simulink model "Simulink_BTL_Model_2018b"  (R2018b)
settings: Solver=ode5  StartTime=0.0  StopTime=300  FixedStep=0.001  RelTol=1e-3
settings Model: Creator=LENOVO  LastModifiedBy=LENOVO
settings DataIOCC: ReturnWorkspaceOutputs=on
settings DebuggingCC: UnconnectedInputMsg=none  UnconnectedOutputMsg=none  UnconnectedLineMsg=none
settings ModelReferenceCC: EnableRefExpFcnMdlSchedulingChecks=off
settings RTWCC: Description=Generic Real-Time Target
settings ConfigComp: CovBoundaryAbsTol=1.0e-5

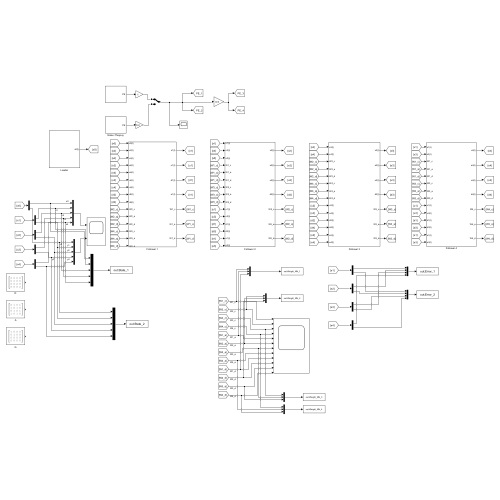
[thumbnail: Simulink's stored preview of the top-level diagram]
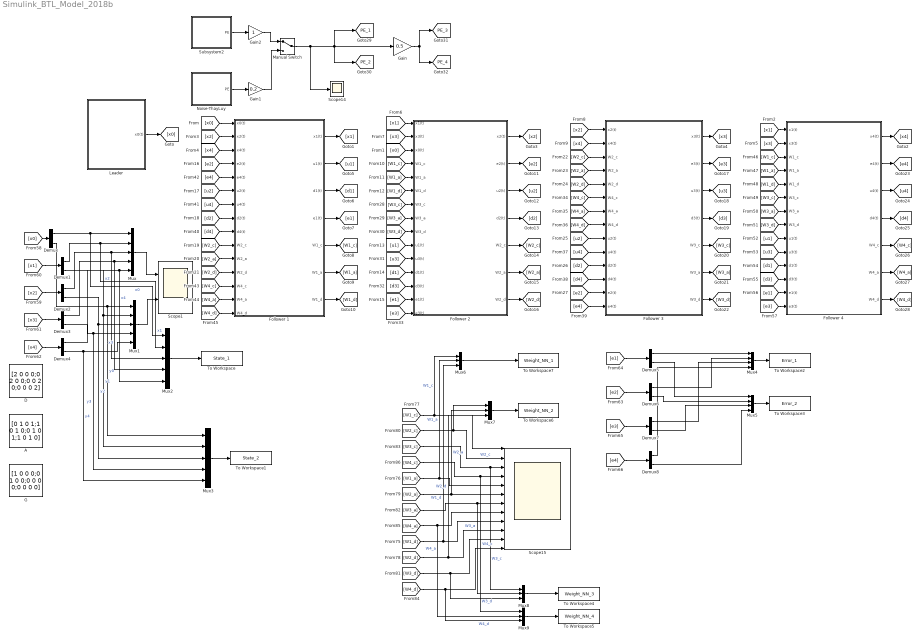
== system Simulink_BTL_Model_2018b ==
  A : Constant  Value=[0 1 0 1;1 0 1 0;0 1 0 1;1 0 1 0]
  D : Constant  Value=[2 0 0 0;0 2 0 0;0 0 2 0;0 0 0 2]
  Demux{,1..8} (9 alike) : Demux  Outputs=2
  Follower 1 : Subsystem
  Follower 2 : Subsystem
  Follower 3 : Subsystem
  Follower 4 : Subsystem
  G : Constant  Value=[1 0 0 0;0 1 0 0;0 0 0 0;0 0 0 0]
  Gain : Gain  Gain=0.5
  Gain1 : Gain  Gain=0.2
  Gain2 : Gain
  Leader : Subsystem
  Manual Switch : ManualSwitch
  Mux{,1..3} (4 alike) : Mux  Inputs=5
  Mux4 : Mux
  Mux5 : Mux
  Mux{6..9} (4 alike) : Mux  Inputs=3
  Noise-ThayLuy : Subsystem
  Scope1 : Scope  NumInputPorts=2
  Scope14 : Scope
  Scope15 : Scope  NumInputPorts=12
  Subsystem2 : Subsystem
  To Workspace : ToWorkspace  VariableName=State_1  SaveFormat=Timeseries  SampleTime=-1
  To Workspace1 : ToWorkspace  VariableName=State_2  SaveFormat=Timeseries  SampleTime=-1
  To Workspace2 : ToWorkspace  VariableName=Error_1  SaveFormat=Timeseries  SampleTime=-1
  To Workspace3 : ToWorkspace  VariableName=Error_2  SaveFormat=Timeseries  SampleTime=-1
  To Workspace4 : ToWorkspace  VariableName=Weight_NN_3  SaveFormat=Timeseries  SampleTime=-1
  To Workspace5 : ToWorkspace  VariableName=Weight_NN_4  SaveFormat=Timeseries  SampleTime=-1
  To Workspace6 : ToWorkspace  VariableName=Weight_NN_2  SaveFormat=Timeseries  SampleTime=-1
  To Workspace7 : ToWorkspace  VariableName=Weight_NN_1  SaveFormat=Timeseries  SampleTime=-1
  tag scope: PE_1=global, PE_2=global, PE_3=global, PE_4=global
  wires:
  Leader/1(x0(t)) -> [x0]
  [x0] -> Follower 1/1(x0(t))
  [x0] -> Follower 2/3(x0(t))
  Follower 1/1(x1(t)) -> [x1]
  [x1] -> Follower 4/1(x1(t))
  Follower 4/1(x4(t)) -> [x4]
  Follower 2/1(x2(t)) -> [x2]
  Follower 3/1(x3(t)) -> [x3]
  [x2] -> Follower 1/2(x2(t))
  [x4] -> Follower 1/3(x4(t))
  [x3] -> Follower 4/2(x3(t))
  [x1] -> Follower 2/1(x1(t))
  [x3] -> Follower 2/2(x3(t))
  [x2] -> Follower 3/1(x2(t))
  [x4] -> Follower 3/2(x4(t))
  Follower 1/2(u1(t)) -> [u1]
  Follower 1/3(d1(t)) -> [d1]
  Follower 1/4(e1(t)) -> [e1]
  Follower 1/5(W1_c) -> [W1_c]
  Follower 1/6(W1_a) -> [W1_a]
  Follower 1/7(W1_d) -> [W1_d]
  [W1_c] -> Follower 2/4(W1_c)
  [W1_a] -> Follower 2/5(W1_a)
  [W1_d] -> Follower 2/6(W1_d)
  [u1] -> Follower 2/10(u1(t))
  [d1] -> Follower 2/12(d1(t))
  [e1] -> Follower 2/14(e1(t))
  Follower 2/2(e2(t)) -> [e2]
  Follower 2/3(u2(t)) -> [u2]
  Follower 2/4(d2(t)) -> [d2]
  Follower 2/5(W2_c) -> [W2_c]
  Follower 2/6(W2_a) -> [W2_a]
  Follower 2/7(W2_d) -> [W2_d]
  [e2] -> Follower 1/4(e2(t))
  [u2] -> Follower 1/6(u2(t))
  [d2] -> Follower 1/8(d2(t))
  [W2_c] -> Follower 1/10(W2_c)
  [W2_a] -> Follower 1/11(W2_a)
  [W2_d] -> Follower 1/12(W2_d)
  Follower 3/2(e3(t)) -> [e3]
  Follower 3/3(u3(t)) -> [u3]
  Follower 3/4(d3(t)) -> [d3]
  Follower 3/5(W3_c) -> [W3_c]
  Follower 3/6(W3_a) -> [W3_a]
  Follower 3/7(W3_d) -> [W3_d]
  [W2_c] -> Follower 3/3(W2_c)
  [W2_a] -> Follower 3/4(W2_a)
  [W2_d] -> Follower 3/5(W2_d)
  [u2] -> Follower 3/9(u2(t))
  [d2] -> Follower 3/11(d2(t))
  [e2] -> Follower 3/13(e2(t))
  [W3_c] -> Follower 2/7(W3_c)
  [W3_a] -> Follower 2/8(W3_a)
  [W3_d] -> Follower 2/9(W3_d)
  [u3] -> Follower 2/11(u3(t))
  [d3] -> Follower 2/13(d3(t))
  [e3] -> Follower 2/15(e3(t))
  Follower 4/2(e4(t)) -> [e4]
  Follower 4/3(u4(t)) -> [u4]
  Follower 4/4(d4(t)) -> [d4]
  Follower 4/5(W4_c) -> [W4_c]
  Follower 4/6(W4_a) -> [W4_a]
  Follower 4/7(W4_d) -> [W4_d]
  [W4_c] -> Follower 3/6(W4_c)
  [W4_a] -> Follower 3/7(W4_a)
  [W4_d] -> Follower 3/8(W4_d)
  [u4] -> Follower 3/10(u4(t))
  [d4] -> Follower 3/12(d4(t))
  [e4] -> Follower 3/14(e4(t))
  [d4] -> Follower 1/9(d4(t))
  [u4] -> Follower 1/7(u4(t))
  [e4] -> Follower 1/5(e4(t))
  [W4_c] -> Follower 1/13(W4_c)
  [W4_a] -> Follower 1/14(W4_a)
  [W4_d] -> Follower 1/15(W4_d)
  [W1_c] -> Follower 4/3(W1_c)
  [W1_a] -> Follower 4/4(W1_a)
  [W1_d] -> Follower 4/5(W1_d)
  [W3_c] -> Follower 4/6(W3_c)
  [W3_a] -> Follower 4/7(W3_a)
  [W3_d] -> Follower 4/8(W3_d)
  [u1] -> Follower 4/9(u1(t))
  [u3] -> Follower 4/10(u3(t))
  [d1] -> Follower 4/11(d1(t))
  [d3] -> Follower 4/12(d3(t))
  [e1] -> Follower 4/13(e1(t))
  [e3] -> Follower 4/14(e3(t))
  [x0] -> Demux/1
  [x1] -> Demux1/1
  [x2] -> Demux2/1
  [x3] -> Demux3/1
  [x4] -> Demux4/1
  Demux/1 -> Mux2/1, Mux/1  "x0"
  Demux1/1 -> Mux2/2, Mux/2  "x1"
  Demux2/1 -> Mux2/3, Mux/3  "x2"
  Demux3/1 -> Mux2/4, Mux/4  "x3"
  Demux4/1 -> Mux2/5, Mux/5  "x4"
  Demux/2 -> Mux3/1, Mux1/1  "y0"
  Demux1/2 -> Mux3/2, Mux1/2  "y1"
  Demux2/2 -> Mux3/3, Mux1/3  "y2"
  Demux3/2 -> Mux3/4, Mux1/4  "y3"
  Demux4/2 -> Mux3/5, Mux1/5  "y4"
  Subsystem2/1(PE) -> Gain2/1
  Gain/1 -> [PE_3], [PE_4]
  Noise-ThayLuy/1(PE) -> Gain1/1
  Manual Switch/1 -> Scope14/1, [PE_1], Gain/1, [PE_2]
  Gain1/1 -> Manual Switch/2
  Gain2/1 -> Manual Switch/1
  [W1_c] -> Mux6/1, Scope15/1  "W1_c"
  [W2_c] -> Mux7/1, Scope15/2  "W2_c"
  [W3_c] -> Mux8/1, Scope15/3  "W3_c"
  [W4_c] -> Mux9/1, Scope15/4  "W4_c"
  [W1_a] -> Mux6/2, Scope15/5  "W1_a"
  [W2_a] -> Mux7/2, Scope15/6  "W2_a"
  [W3_a] -> Mux8/2, Scope15/7  "W3_a"
  [W4_a] -> Mux9/2, Scope15/8  "W4_a"
  [W1_d] -> Mux6/3, Scope15/9  "W1_d"
  [W2_d] -> Scope15/10, Mux7/3  "W2_d"
  [W3_d] -> Mux8/3, Scope15/11  "W3_d"
  [W4_d] -> Mux9/3, Scope15/12  "W4_d"
  Mux/1 -> Scope1/1
  Mux1/1 -> Scope1/2
  Mux2/1 -> To Workspace/1
  Mux3/1 -> To Workspace1/1
  [e1] -> Demux5/1
  [e2] -> Demux6/1
  [e3] -> Demux7/1
  [e4] -> Demux8/1
  Demux5/1 -> Mux4/1
  Demux6/1 -> Mux4/2
  Demux7/1 -> Mux4/3
  Demux8/1 -> Mux4/4
  Demux5/2 -> Mux5/1
  Demux6/2 -> Mux5/2
  Demux7/2 -> Mux5/3
  Demux8/2 -> Mux5/4
  Mux4/1 -> To Workspace2/1
  Mux5/1 -> To Workspace3/1
  Mux8/1 -> To Workspace4/1
  Mux9/1 -> To Workspace5/1
  Mux7/1 -> To Workspace6/1
  Mux6/1 -> To Workspace7/1

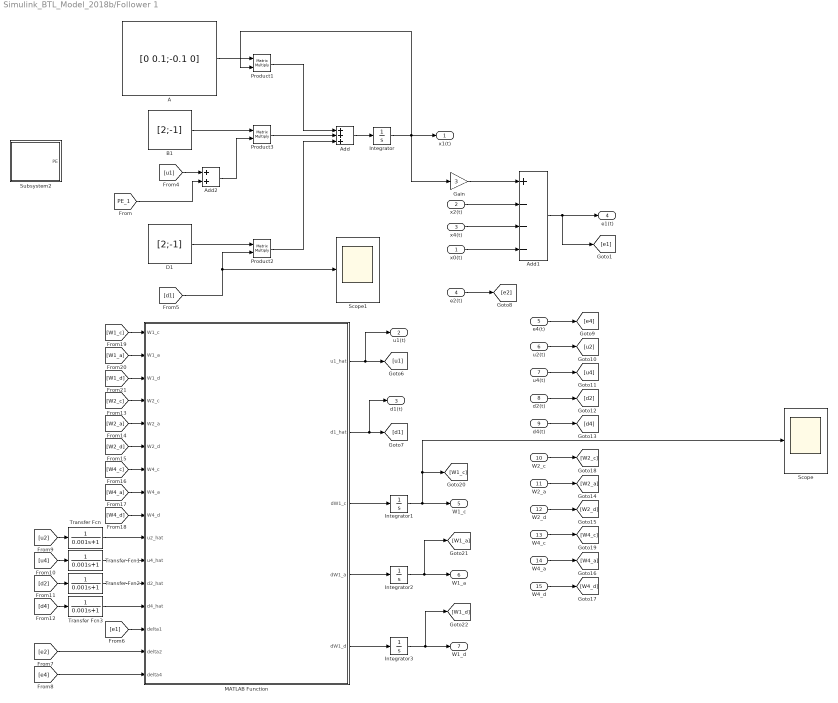
== system Simulink_BTL_Model_2018b/Follower 1 ==
  x0(t) : Inport
  x2(t) : Inport  Port=2
  x4(t) : Inport  Port=3
  e2(t) : Inport  Port=4
  e4(t) : Inport  Port=5
  u2(t) : Inport  Port=6
  u4(t) : Inport  Port=7
  d2(t) : Inport  Port=8
  d4(t) : Inport  Port=9
  W2_c : Inport  Port=10
  W2_a : Inport  Port=11
  W2_d : Inport  Port=12
  W4_c : Inport  Port=13
  W4_a : Inport  Port=14
  W4_d : Inport  Port=15
  A : Constant  Value=[0 0.1;-0.1 0]
  Add : Sum  Inputs=+++
  Add1 : Sum  Inputs=+---
  Add2 : Sum
  B1 : Constant  Value=[2;-1]  VectorParams1D=off
  D1 : Constant  Value=[2;-1]  VectorParams1D=off
  Gain : Gain  Gain=3
  Integrator : Integrator  InitialCondition=[1;0]
  Integrator1 : Integrator
  Integrator2 : Integrator
  Integrator3 : Integrator
  MATLAB Function : MATLAB Function  TreatAsAtomicUnit=on
  Product1 : Product  Multiplication=Matrix(*)
  Product2 : Product  Multiplication=Matrix(*)
  Product3 : Product  Multiplication=Matrix(*)
  Scope : Scope
  Scope1 : Scope
  Subsystem2 : Subsystem
  Transfer Fcn{,1..3} (4 alike) : TransferFcn  Denominator=[0.001 1]
  x1(t) : Outport
  u1(t) : Outport  Port=2
  d1(t) : Outport  Port=3
  e1(t) : Outport  Port=4
  W1_c : Outport  Port=5
  W1_a : Outport  Port=6
  W1_d : Outport  Port=7
  wires:
  A/1 -> Product1/1
  Product1/1 -> Add/1
  D1/1 -> Product2/1
  Add/1 -> Integrator/1
  Integrator/1 -> Gain/1, Product1/2, x1(t)/1
  B1/1 -> Product3/1
  Product3/1 -> Add/2
  Product2/1 -> Add/3
  x2(t)/1 -> Add1/2
  x4(t)/1 -> Add1/3
  x0(t)/1 -> Add1/4
  Gain/1 -> Add1/1
  Add1/1 -> [e1], e1(t)/1
  MATLAB Function/3(dW1_c) -> Integrator1/1
  MATLAB Function/4(dW1_a) -> Integrator2/1
  MATLAB Function/5(dW1_d) -> Integrator3/1
  MATLAB Function/1(u1_hat) -> u1(t)/1, [u1]
  MATLAB Function/2(d1_hat) -> d1(t)/1, [d1]
  [d1] -> Scope1/1, Product2/2
  [u1] -> Add2/1
  Add2/1 -> Product3/2
  [e1] -> MATLAB Function/14(delta1)
  e2(t)/1 -> [e2]
  e4(t)/1 -> [e4]
  u2(t)/1 -> [u2]
  u4(t)/1 -> [u4]
  d2(t)/1 -> [d2]
  d4(t)/1 -> [d4]
  [u2] -> Transfer Fcn/1
  [u4] -> Transfer Fcn1/1
  [d2] -> Transfer Fcn2/1
  [d4] -> Transfer Fcn3/1
  W2_d/1 -> [W2_d]
  W2_a/1 -> [W2_a]
  W2_c/1 -> [W2_c]
  W4_a/1 -> [W4_a]
  W4_c/1 -> [W4_c]
  W4_d/1 -> [W4_d]
  [W2_c] -> MATLAB Function/4(W2_c)
  [W2_a] -> MATLAB Function/5(W2_a)
  [W2_d] -> MATLAB Function/6(W2_d)
  [W4_c] -> MATLAB Function/7(W4_c)
  [W4_a] -> MATLAB Function/8(W4_a)
  [W4_d] -> MATLAB Function/9(W4_d)
  Integrator1/1 -> Scope/1, [W1_c], W1_c/1
  Integrator2/1 -> [W1_a], W1_a/1
  Integrator3/1 -> [W1_d], W1_d/1
  [W1_c] -> MATLAB Function/1(W1_c)
  [W1_a] -> MATLAB Function/2(W1_a)
  [W1_d] -> MATLAB Function/3(W1_d)
  Transfer Fcn/1 -> MATLAB Function/10(u2_hat)
  Transfer Fcn1/1 -> MATLAB Function/11(u4_hat)
  Transfer Fcn2/1 -> MATLAB Function/12(d2_hat)
  Transfer Fcn3/1 -> MATLAB Function/13(d4_hat)
  [e2] -> MATLAB Function/15(delta2)
  [e4] -> MATLAB Function/16(delta4)
  [PE_1] -> Add2/2

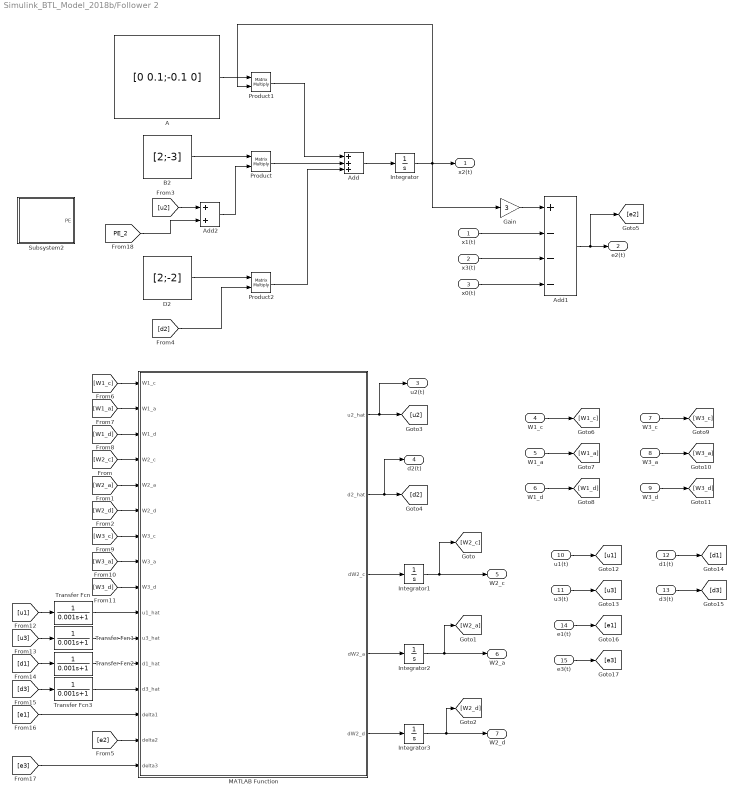
== system Simulink_BTL_Model_2018b/Follower 2 ==
  x1(t) : Inport
  x3(t) : Inport  Port=2
  x0(t) : Inport  Port=3
  W1_c : Inport  Port=4
  W1_a : Inport  Port=5
  W1_d : Inport  Port=6
  W3_c : Inport  Port=7
  W3_a : Inport  Port=8
  W3_d : Inport  Port=9
  u1(t) : Inport  Port=10
  u3(t) : Inport  Port=11
  d1(t) : Inport  Port=12
  d3(t) : Inport  Port=13
  e1(t) : Inport  Port=14
  e3(t) : Inport  Port=15
  A : Constant  Value=[0 0.1;-0.1 0]
  Add : Sum  Inputs=+++
  Add1 : Sum  Inputs=+---
  Add2 : Sum
  B2 : Constant  Value=[2;-3]  VectorParams1D=off
  D2 : Constant  Value=[2;-2]  VectorParams1D=off
  Gain : Gain  Gain=3
  Integrator : Integrator  InitialCondition=[1;0]
  Integrator1 : Integrator
  Integrator2 : Integrator
  Integrator3 : Integrator
  MATLAB Function : MATLAB Function  TreatAsAtomicUnit=on
  Product : Product  Multiplication=Matrix(*)
  Product1 : Product  Multiplication=Matrix(*)
  Product2 : Product  Multiplication=Matrix(*)
  Subsystem2 : Subsystem
  Transfer Fcn{,1..3} (4 alike) : TransferFcn  Denominator=[0.001 1]
  x2(t) : Outport
  e2(t) : Outport  Port=2
  u2(t) : Outport  Port=3
  d2(t) : Outport  Port=4
  W2_c : Outport  Port=5
  W2_a : Outport  Port=6
  W2_d : Outport  Port=7
  wires:
  Integrator/1 -> Gain/1, x2(t)/1, Product1/2
  Product1/1 -> Add/1
  Add/1 -> Integrator/1
  B2/1 -> Product/1
  A/1 -> Product1/1
  Product/1 -> Add/2
  D2/1 -> Product2/1
  Product2/1 -> Add/3
  Add1/1 -> [e2], e2(t)/1
  x1(t)/1 -> Add1/2
  x3(t)/1 -> Add1/3
  x0(t)/1 -> Add1/4
  Gain/1 -> Add1/1
  MATLAB Function/3(dW2_c) -> Integrator1/1
  MATLAB Function/4(dW2_a) -> Integrator2/1
  MATLAB Function/5(dW2_d) -> Integrator3/1
  Integrator1/1 -> W2_c/1, [W2_c]
  [W2_c] -> MATLAB Function/4(W2_c)
  Integrator2/1 -> W2_a/1, [W2_a]
  [W2_a] -> MATLAB Function/5(W2_a)
  [W2_d] -> MATLAB Function/6(W2_d)
  Integrator3/1 -> [W2_d], W2_d/1
  MATLAB Function/1(u2_hat) -> u2(t)/1, [u2]
  MATLAB Function/2(d2_hat) -> d2(t)/1, [d2]
  [u2] -> Add2/1
  Add2/1 -> Product/2
  [d2] -> Product2/2
  [e2] -> MATLAB Function/15(delta2)
  W1_c/1 -> [W1_c]
  W1_a/1 -> [W1_a]
  W1_d/1 -> [W1_d]
  W3_d/1 -> [W3_d]
  W3_c/1 -> [W3_c]
  W3_a/1 -> [W3_a]
  u1(t)/1 -> [u1]
  u3(t)/1 -> [u3]
  d3(t)/1 -> [d3]
  d1(t)/1 -> [d1]
  e1(t)/1 -> [e1]
  e3(t)/1 -> [e3]
  [W1_c] -> MATLAB Function/1(W1_c)
  [W1_d] -> MATLAB Function/3(W1_d)
  [W3_c] -> MATLAB Function/7(W3_c)
  [W3_a] -> MATLAB Function/8(W3_a)
  [W3_d] -> MATLAB Function/9(W3_d)
  [u1] -> Transfer Fcn/1
  [u3] -> Transfer Fcn1/1
  [d1] -> Transfer Fcn2/1
  [W1_a] -> MATLAB Function/2(W1_a)
  [d3] -> Transfer Fcn3/1
  Transfer Fcn/1 -> MATLAB Function/10(u1_hat)
  Transfer Fcn1/1 -> MATLAB Function/11(u3_hat)
  Transfer Fcn2/1 -> MATLAB Function/12(d1_hat)
  Transfer Fcn3/1 -> MATLAB Function/13(d3_hat)
  [e1] -> MATLAB Function/14(delta1)
  [e3] -> MATLAB Function/16(delta3)
  [PE_2] -> Add2/2

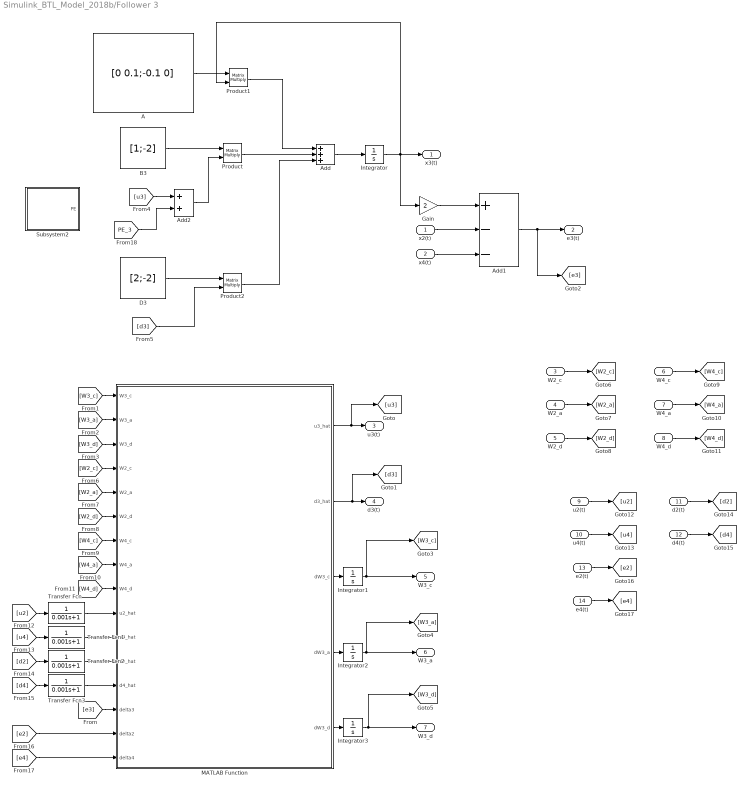
== system Simulink_BTL_Model_2018b/Follower 3 ==
  x2(t) : Inport
  x4(t) : Inport  Port=2
  W2_c : Inport  Port=3
  W2_a : Inport  Port=4
  W2_d : Inport  Port=5
  W4_c : Inport  Port=6
  W4_a : Inport  Port=7
  W4_d : Inport  Port=8
  u2(t) : Inport  Port=9
  u4(t) : Inport  Port=10
  d2(t) : Inport  Port=11
  d4(t) : Inport  Port=12
  e2(t) : Inport  Port=13
  e4(t) : Inport  Port=14
  A : Constant  Value=[0 0.1;-0.1 0]
  Add : Sum  Inputs=+++
  Add1 : Sum  Inputs=+--
  Add2 : Sum
  B3 : Constant  Value=[1;-2]  VectorParams1D=off
  D3 : Constant  Value=[2;-2]  VectorParams1D=off
  Gain : Gain  Gain=2
  Integrator : Integrator  InitialCondition=[1;0]
  Integrator1 : Integrator
  Integrator2 : Integrator
  Integrator3 : Integrator
  MATLAB Function : MATLAB Function  TreatAsAtomicUnit=on
  Product : Product  Multiplication=Matrix(*)
  Product1 : Product  Multiplication=Matrix(*)
  Product2 : Product  Multiplication=Matrix(*)
  Subsystem2 : Subsystem
  Transfer Fcn{,1..3} (4 alike) : TransferFcn  Denominator=[0.001 1]
  x3(t) : Outport
  e3(t) : Outport  Port=2
  u3(t) : Outport  Port=3
  d3(t) : Outport  Port=4
  W3_c : Outport  Port=5
  W3_a : Outport  Port=6
  W3_d : Outport  Port=7
  wires:
  Integrator/1 -> Gain/1, x3(t)/1, Product1/2
  Product1/1 -> Add/1
  Add/1 -> Integrator/1
  B3/1 -> Product/1
  A/1 -> Product1/1
  Product/1 -> Add/2
  D3/1 -> Product2/1
  Product2/1 -> Add/3
  x2(t)/1 -> Add1/2
  Gain/1 -> Add1/1
  x4(t)/1 -> Add1/3
  Add1/1 -> [e3], e3(t)/1
  MATLAB Function/1(u3_hat) -> [u3], u3(t)/1
  MATLAB Function/2(d3_hat) -> d3(t)/1, [d3]
  MATLAB Function/3(dW3_c) -> Integrator1/1
  MATLAB Function/4(dW3_a) -> Integrator2/1
  MATLAB Function/5(dW3_d) -> Integrator3/1
  [e3] -> MATLAB Function/14(delta3)
  [W3_c] -> MATLAB Function/1(W3_c)
  [W3_a] -> MATLAB Function/2(W3_a)
  [W3_d] -> MATLAB Function/3(W3_d)
  [u3] -> Add2/1
  Add2/1 -> Product/2
  [d3] -> Product2/2
  e2(t)/1 -> [e2]
  W4_c/1 -> [W4_c]
  W4_d/1 -> [W4_d]
  W4_a/1 -> [W4_a]
  W2_d/1 -> [W2_d]
  u2(t)/1 -> [u2]
  W2_c/1 -> [W2_c]
  W2_a/1 -> [W2_a]
  d4(t)/1 -> [d4]
  d2(t)/1 -> [d2]
  e4(t)/1 -> [e4]
  u4(t)/1 -> [u4]
  [W2_c] -> MATLAB Function/4(W2_c)
  [W2_a] -> MATLAB Function/5(W2_a)
  [W2_d] -> MATLAB Function/6(W2_d)
  [W4_c] -> MATLAB Function/7(W4_c)
  [W4_a] -> MATLAB Function/8(W4_a)
  [W4_d] -> MATLAB Function/9(W4_d)
  [u2] -> Transfer Fcn/1
  [u4] -> Transfer Fcn1/1
  [d2] -> Transfer Fcn2/1
  [d4] -> Transfer Fcn3/1
  Transfer Fcn/1 -> MATLAB Function/10(u2_hat)
  Transfer Fcn1/1 -> MATLAB Function/11(u4_hat)
  Transfer Fcn2/1 -> MATLAB Function/12(d2_hat)
  Transfer Fcn3/1 -> MATLAB Function/13(d4_hat)
  [e2] -> MATLAB Function/15(delta2)
  [e4] -> MATLAB Function/16(delta4)
  Integrator1/1 -> [W3_c], W3_c/1
  Integrator2/1 -> [W3_a], W3_a/1
  Integrator3/1 -> [W3_d], W3_d/1
  [PE_3] -> Add2/2

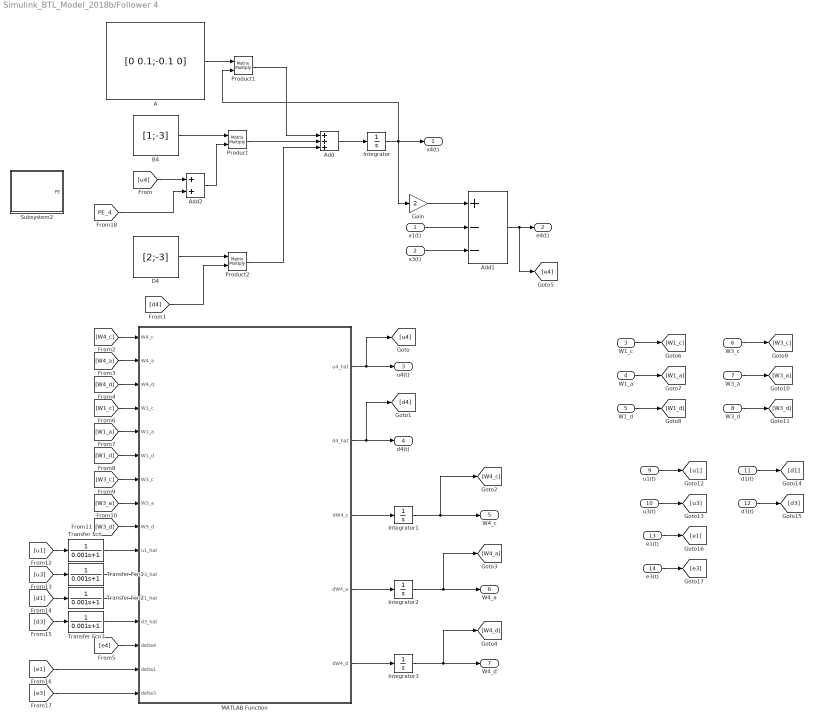
== system Simulink_BTL_Model_2018b/Follower 4 ==
  x1(t) : Inport
  x3(t) : Inport  Port=2
  W1_c : Inport  Port=3
  W1_a : Inport  Port=4
  W1_d : Inport  Port=5
  W3_c : Inport  Port=6
  W3_a : Inport  Port=7
  W3_d : Inport  Port=8
  u1(t) : Inport  Port=9
  u3(t) : Inport  Port=10
  d1(t) : Inport  Port=11
  d3(t) : Inport  Port=12
  e1(t) : Inport  Port=13
  e3(t) : Inport  Port=14
  A : Constant  Value=[0 0.1;-0.1 0]
  Add : Sum  Inputs=+++
  Add1 : Sum  Inputs=+--
  Add2 : Sum
  B4 : Constant  Value=[1;-3]  VectorParams1D=off
  D4 : Constant  Value=[2;-3]  VectorParams1D=off
  Gain : Gain  Gain=2
  Integrator : Integrator  InitialCondition=[1;0]
  Integrator1 : Integrator
  Integrator2 : Integrator
  Integrator3 : Integrator
  MATLAB Function : MATLAB Function  TreatAsAtomicUnit=on
  Product : Product  Multiplication=Matrix(*)
  Product1 : Product  Multiplication=Matrix(*)
  Product2 : Product  Multiplication=Matrix(*)
  Subsystem2 : Subsystem
  Transfer Fcn{,1..3} (4 alike) : TransferFcn  Denominator=[0.001 1]
  x4(t) : Outport
  e4(t) : Outport  Port=2
  u4(t) : Outport  Port=3
  d4(t) : Outport  Port=4
  W4_c : Outport  Port=5
  W4_a : Outport  Port=6
  W4_d : Outport  Port=7
  wires:
  Product1/1 -> Add/1
  B4/1 -> Product/1
  A/1 -> Product1/1
  Product/1 -> Add/2
  D4/1 -> Product2/1
  Product2/1 -> Add/3
  Add/1 -> Integrator/1
  Integrator/1 -> Product1/2, Gain/1, x4(t)/1
  Add1/1 -> [e4], e4(t)/1
  x1(t)/1 -> Add1/2
  x3(t)/1 -> Add1/3
  Gain/1 -> Add1/1
  MATLAB Function/1(u4_hat) -> [u4], u4(t)/1
  MATLAB Function/2(d4_hat) -> [d4], d4(t)/1
  [u4] -> Add2/1
  [d4] -> Product2/2
  MATLAB Function/3(dW4_c) -> Integrator1/1
  MATLAB Function/4(dW4_a) -> Integrator2/1
  MATLAB Function/5(dW4_d) -> Integrator3/1
  Integrator1/1 -> [W4_c], W4_c/1
  Integrator2/1 -> [W4_a], W4_a/1
  Integrator3/1 -> [W4_d], W4_d/1
  [W4_c] -> MATLAB Function/1(W4_c)
  [W4_a] -> MATLAB Function/2(W4_a)
  [W4_d] -> MATLAB Function/3(W4_d)
  [e4] -> MATLAB Function/14(delta4)
  u3(t)/1 -> [u3]
  e3(t)/1 -> [e3]
  d1(t)/1 -> [d1]
  W1_c/1 -> [W1_c]
  u1(t)/1 -> [u1]
  d3(t)/1 -> [d3]
  W1_a/1 -> [W1_a]
  W3_a/1 -> [W3_a]
  W3_c/1 -> [W3_c]
  e1(t)/1 -> [e1]
  W3_d/1 -> [W3_d]
  W1_d/1 -> [W1_d]
  [W1_c] -> MATLAB Function/4(W1_c)
  [W1_a] -> MATLAB Function/5(W1_a)
  [W1_d] -> MATLAB Function/6(W1_d)
  [W3_c] -> MATLAB Function/7(W3_c)
  [W3_a] -> MATLAB Function/8(W3_a)
  [W3_d] -> MATLAB Function/9(W3_d)
  [u1] -> Transfer Fcn/1
  [u3] -> Transfer Fcn1/1
  [d1] -> Transfer Fcn2/1
  [d3] -> Transfer Fcn3/1
  Add2/1 -> Product/2
  Transfer Fcn/1 -> MATLAB Function/10(u1_hat)
  Transfer Fcn1/1 -> MATLAB Function/11(u3_hat)
  Transfer Fcn2/1 -> MATLAB Function/12(d1_hat)
  Transfer Fcn3/1 -> MATLAB Function/13(d3_hat)
  [e1] -> MATLAB Function/15(delta1)
  [e3] -> MATLAB Function/16(delta3)
  [PE_4] -> Add2/2

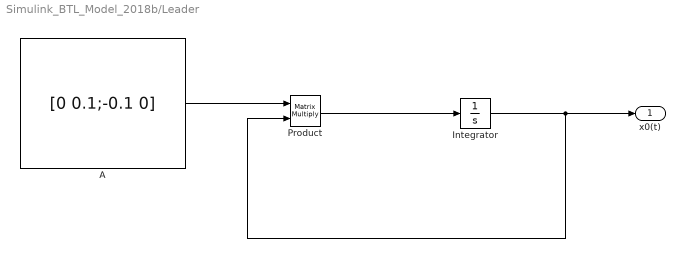
== system Simulink_BTL_Model_2018b/Leader ==
  A : Constant  Value=[0 0.1;-0.1 0]
  Integrator : Integrator  InitialCondition=[1;0]
  Product : Product  Multiplication=Matrix(*)
  x0(t) : Outport
  wires:
  Product/1 -> Integrator/1
  A/1 -> Product/1
  Integrator/1 -> x0(t)/1, Product/2

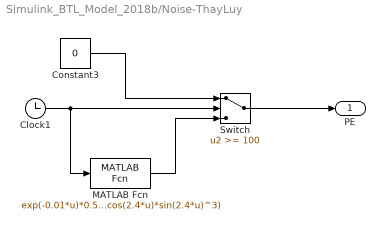
== system Simulink_BTL_Model_2018b/Noise-ThayLuy ==
  Clock1 : Clock
  Constant3 : Constant  Value=0
  MATLAB Fcn : MATLABFcn  MATLABFcn=exp(-0.01*u)*0.5*(sin(u)^2*cos(u)+sin(2*u)^2*cos(0.1*u)+sin(-1.2*u)^2*cos(0.5*u)+sin(u)^5+sin(1.12*u)^2+cos(2.4*u)*sin(2.4*u)^3)
  Switch : Switch  Threshold=100
  PE : Outport
  wires:
  Constant3/1 -> Switch/1
  Clock1/1 -> Switch/2, MATLAB Fcn/1
  MATLAB Fcn/1 -> Switch/3
  Switch/1 -> PE/1

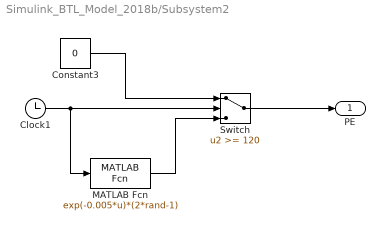
== system Simulink_BTL_Model_2018b/Subsystem2 ==
  Clock1 : Clock
  Constant3 : Constant  Value=0
  MATLAB Fcn : MATLABFcn  MATLABFcn=exp(-0.005*u)*(2*rand-1)
  Switch : Switch  Threshold=120
  PE : Outport
  wires:
  Constant3/1 -> Switch/1
  Clock1/1 -> Switch/2, MATLAB Fcn/1
  MATLAB Fcn/1 -> Switch/3
  Switch/1 -> PE/1

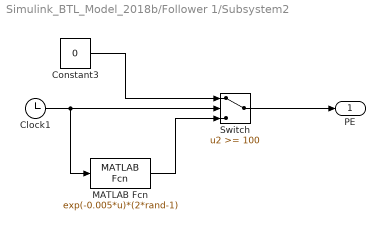
== system Simulink_BTL_Model_2018b/Follower 1/Subsystem2 ==
  Clock1 : Clock
  Constant3 : Constant  Value=0
  MATLAB Fcn : MATLABFcn  MATLABFcn=exp(-0.005*u)*(2*rand-1)
  Switch : Switch  Threshold=100
  PE : Outport
  wires:
  Constant3/1 -> Switch/1
  Clock1/1 -> Switch/2, MATLAB Fcn/1
  MATLAB Fcn/1 -> Switch/3
  Switch/1 -> PE/1

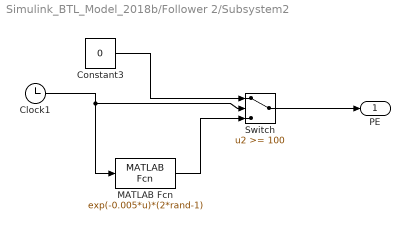
== system Simulink_BTL_Model_2018b/Follower 2/Subsystem2 ==
  Clock1 : Clock
  Constant3 : Constant  Value=0
  MATLAB Fcn : MATLABFcn  MATLABFcn=exp(-0.005*u)*(2*rand-1)
  Switch : Switch  Threshold=100
  PE : Outport
  wires:
  Constant3/1 -> Switch/1
  Clock1/1 -> Switch/2, MATLAB Fcn/1
  MATLAB Fcn/1 -> Switch/3
  Switch/1 -> PE/1

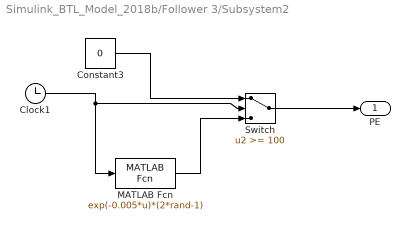
== system Simulink_BTL_Model_2018b/Follower 3/Subsystem2 ==
  Clock1 : Clock
  Constant3 : Constant  Value=0
  MATLAB Fcn : MATLABFcn  MATLABFcn=exp(-0.005*u)*(2*rand-1)
  Switch : Switch  Threshold=100
  PE : Outport
  wires:
  Constant3/1 -> Switch/1
  Clock1/1 -> Switch/2, MATLAB Fcn/1
  MATLAB Fcn/1 -> Switch/3
  Switch/1 -> PE/1

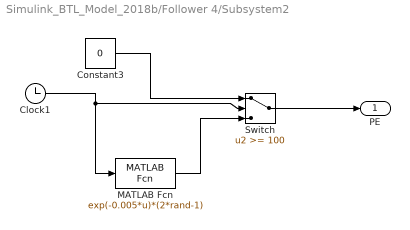
== system Simulink_BTL_Model_2018b/Follower 4/Subsystem2 ==
  Clock1 : Clock
  Constant3 : Constant  Value=0
  MATLAB Fcn : MATLABFcn  MATLABFcn=exp(-0.005*u)*(2*rand-1)
  Switch : Switch  Threshold=100
  PE : Outport
  wires:
  Constant3/1 -> Switch/1
  Clock1/1 -> Switch/2, MATLAB Fcn/1
  MATLAB Fcn/1 -> Switch/3
  Switch/1 -> PE/1

== matlab function Simulink_BTL_Model_2018b/Follower 2/MATLAB Function ==
  data: u2_hat output; W1_c input; W1_a input; W1_d input; W2_c input; W2_a input; W2_d input; W3_c input; W3_a input; W3_d input; u1_hat input; u3_hat input; d1_hat input; d3_hat input; delta1 input; delta2 input; delta3 input; d2_hat output; dW2_c output; dW2_a output; dW2_d output
function [u2_hat, d2_hat, dW2_c, dW2_a, dW2_d] = Follower2_Controller( W1_c, W1_a, W1_d, W2_c, W2_a, W2_d, W3_c, W3_a, W3_d, u1_hat, u3_hat, d1_hat, d3_hat,delta1, delta2, delta3)
    % CÁC BIẾN ĐẦU VÀO TỪ SIMULINK:
    % x1, x0, x2, x4: Trạng thái của bản thân, leader và hàng xóm (2x1)
    % W1_*, W2_*, W4_*: Trọng số của 3 mạng NNs của bản thân và hàng xóm (3x1)
    % u1_hat, u3_hat, d1_hat, d3_hat: Tín hiệu điều khiển/nhiễu của hàng xóm (1x1)
    % delta1, delta3: Sai số bám sát của hàng xóm (2x1)
    u2_hat = zeros(1,1);
    d2_hat = zeros(1,1);
    dW2_c = zeros(3,1);
    dW2_a = zeros(3,1);
    dW2_d = zeros(3,1);
    %% 1. KHỞI TẠO THÔNG SỐ HỆ THỐNG VÀ ĐỒ THỊ (Hardcode cho Node 1)
    % Đồ thị: N1 = {1, 3}
    d1 = 2; g1 = 1;
    d2 = 2; g2 = 1;
    d3 = 2; g3 = 0;
    
    gamma = 1; % Hệ số L2-gain (thay đổi theo thiết kế của bạn)
    
    % Ma trận động học (Ví dụ theo bài báo, hãy thay số thực tế của bạn)
    A  = [0 0.1; -0.1 0]; 
    B1 = [2; -1]; D1 = [2; -1];
    B2 = [2; -3]; D2 = [2; -2];
    B3 = [1; -2]; D3 = [2; -2];
    
    % Ma trận trọng số chi phí (Q, R, T)
    Q22 = eye(2);
    R22 = 1; T22 = 1;
    R21 = 1; T21 = 1; % Trọng số cho u1, d1 trong hàm mục tiêu của 1
    R23 = 1; T23 = 1; % Trọng số cho u3, d3 trong hàm mục tiêu của 1
    
    R11 = 1; T11 = 1; % Của node 1
    R33 = 1; T33 = 1; % Của node 3
    
    % Tốc độ học (Learning rates) và tham số mạng NNs
    a2 = 0.005; a2_a = 0.007; a2_d = 0.005;
    S2 = 10; F2 = 10; S_bar2 = 10; F_bar2 = 10;

    % Hàm tính ma trận đạo hàm 3x2
    dphi_1 = [2*delta1(1), 0; 
              delta1(2), delta1(1); 
              0, 2*delta1(2)];
          
    dphi_2 = [2*delta2(1), 0; 
              delta2(2), delta2(1); 
              0, 2*delta2(2)];
          
    dphi_3 = [2*delta3(1), 0; 
              delta3(2), delta3(1); 
              0, 2*delta3(2)];

    %% 3. TÍNH TÍN HIỆU ĐẦU RA ACTOR & DISTURBANCE (Eq 55, 56)
    % Tính tín hiệu u1, v1 dự kiến dựa trên trọng số hiện tại
    u2_hat = -(d2 + g2) * (1/R22) * B2' * dphi_2' * W2_a;
    d2_hat = (1/gamma^2) * (d2 + g2) * (1/T22) * D2' * dphi_2' * W2_d;

    %% 4. TÍNH TOÁN CÁC BIẾN TRUNG GIAN
    % D_bar và E_bar (3x3)
    D_bar2 = dphi_2 * B2 * (1/R22) * B2' * dphi_2';
    E_bar2 = dphi_2 * D2 * (1/T22) * D2' * dphi_2';
    
    % Tính sigma_{i+N} (Lưu ý: dùng u_hat, v_hat theo đúng lý thuyết)
    % sigma_2_N = dphi_2 * (A * delta2 + (d2 + g2)*B2*u3_hat - (B3*u3_hat + B1*u1_hat) ...
    %                       + (d2 + g2)*D2*d3_hat - (D3*d3_hat + D1*d1_hat));

    sigma_2_N = dphi_2 * (A * delta2 + (d2 + g2)*B2*u2_hat - (B3*u3_hat + B1*u1_hat) ...
                          + (d2 + g2)*D2*d2_hat - (D3*d3_hat + D1*d1_hat));
                      
    m_s2 = (sigma_2_N' * sigma_2_N) + 1;
    sigma_bar_2_N = sigma_2_N / m_s2; % Vector 3x1

    %% 5. TÍNH TỔNG TỪ CÁC HÀNG XÓM (Node 2 và Node 4)
    % -- Của Node 1 --
    term_B1 = dphi_1 * B1 * (1/R11) * R21 * (1/R11) * B1' * dphi_1';
    term_D1 = dphi_1 * D1 * (1/T11) * T21 * (1/T11) * D1' * dphi_1';
    
    sum57_a_1 = (d1 + g1)^2 * W1_a' * term_B1 * W1_a;
    sum57_d_1 = (d1 + g1)^2 * W1_d' * term_D1 * W1_d;
    sum58_a_1 = (d1 + g1)^2 * term_B1 * W1_a .* (sigma_bar_2_N' * W1_c / m_s2);
    sum59_d_1 = (d1 + g1)^2 * term_D1 * W1_d .* (sigma_bar_2_N' * W1_c / m_s2);
    
    % -- Của Node 3 --
    term_B3 = dphi_3 * B3 * (1/R33) * R23 * (1/R33) * B3' * dphi_3';
    term_D3 = dphi_3 * D3 * (1/T33) * T23 * (1/T33) * D3' * dphi_3';
    
    sum57_a_3 = (d3 + g3)^2 * W3_a' * term_B3 * W3_a;
    sum57_d_3 = (d3 + g3)^2 * W3_d' * term_D3 * W3_d;
    sum58_a_3 = (d3 + g3)^2 * term_B3 * W3_a .* (sigma_bar_2_N' * W3_c / m_s2);
    sum59_d_3 = (d3 + g3)^2 * term_D3 * W3_d .* (sigma_bar_2_N' * W3_c / m_s2);
    
    % Gộp tổng
    sum57_actor = sum57_a_1 + sum57_a_3; % Vô hướng
    sum57_dist  = sum57_d_1 + sum57_d_3; % Vô hướng
    sum58_actor = sum58_a_1 + sum58_a_3; % Vector 3x1
    sum59_dist  = sum59_d_1 + sum59_d_3; % Vector 3x1

    %% 6. LUẬT CẬP NHẬT TRỌNG SỐ (Equations 57, 58, 59)
    % 6.1 Critic
    term1_57 = sigma_2_N' * W2_c + 0.5 * delta2' * Q22 * delta2;
    term2_57 = 0.5 * (d2 + g2)^2 * W2_a' * D_bar2 * W2_a;
    term3_57 = - (1 / (2 * gamma^2)) * (d2 + g2)^2 * W2_d' * E_bar2 * W2_d;
    term_sum_57 = 0.5 * sum57_actor - (1 / (2 * gamma^2)) * sum57_dist;
    
    gain_57 = a2 * (sigma_2_N / (m_s2^2)); % Vector 3x1
    dW2_c = - gain_57 * (term1_57 + term2_57 + term3_57 + term_sum_57);
    
    % 6.2 Actor
    % term1_58 = S2 * W2_a - F2 * W2_c;
    term1_58 = S2 * W2_a - F2 * ( W2_c) ;  % scalar
    term2_58 = (d2 + g2)^2 * D_bar2 * W2_a .* (sigma_bar_2_N' * W2_c / m_s2);
    dW2_a = - a2_a * (term1_58 - term2_58 - sum58_actor);
    
    % 6.3 Disturbance
    % term1_59 = S_bar2 * W1_d - F_bar2 * W1_c;
    term1_59 = S_bar2 * W2_d - F_bar2 * sigma_bar_2_N * (sigma_bar_2_N' * W2_c);

    term2_59 = (1 / gamma^2) * (d2 + g2)^2 * E_bar2 * W2_d .* (sigma_bar_2_N' * W2_c / m_s2);
    term_sum_59 = (1 / gamma^2) * sum59_dist;
    dW2_d = - a2_d * (term1_59 + term2_59 + term_sum_59);

end

== matlab function Simulink_BTL_Model_2018b/Follower 1/MATLAB Function ==
  data: u1_hat output; W1_c input; W1_a input; W1_d input; W2_c input; W2_a input; W2_d input; W4_c input; W4_a input; W4_d input; u2_hat input; u4_hat input; d2_hat input; d4_hat input; delta1 input; delta2 input; delta4 input; d1_hat output; dW1_c output; dW1_a output; dW1_d output
function [u1_hat, d1_hat, dW1_c, dW1_a, dW1_d] = Follower1_Controller( W1_c, W1_a, W1_d, W2_c, W2_a, W2_d, W4_c, W4_a, W4_d, u2_hat, u4_hat, d2_hat, d4_hat,delta1, delta2, delta4)
    % CÁC BIẾN ĐẦU VÀO TỪ SIMULINK:
    % x1, x0, x2, x4: Trạng thái của bản thân, leader và hàng xóm (2x1)
    % W1_*, W2_*, W4_*: Trọng số của 3 mạng NNs của bản thân và hàng xóm (3x1)
    % u2_hat, u4_hat, v2_hat, v4_hat: Tín hiệu điều khiển/nhiễu của hàng xóm (1x1)
    % delta2, delta4: Sai số bám sát của hàng xóm (2x1)
    u1_hat = zeros(1,1);
    d1_hat = zeros(1,1);
    dW1_c = zeros(3,1);
    dW1_a = zeros(3,1);
    dW1_d = zeros(3,1);
    %% 1. KHỞI TẠO THÔNG SỐ HỆ THỐNG VÀ ĐỒ THỊ (Hardcode cho Node 1)
    % Đồ thị: N1 = {2, 4}
    d1 = 2; g1 = 1;
    d2 = 2; g2 = 1;
    d4 = 2; g4 = 0;
    
    gamma = 1; % Hệ số L2-gain (thay đổi theo thiết kế của bạn)
    
    % Ma trận động học (Ví dụ theo bài báo, hãy thay số thực tế của bạn)
    A  = [0 0.1; -0.1 0]; 
    B1 = [2; -1]; D1 = [2; -1];
    B2 = [2; -3]; D2 = [2; -2];
    B4 = [1; -3]; D4 = [2; -3];
    
    % Ma trận trọng số chi phí (Q, R, T)
    Q11 = eye(2);
    R11 = 1; T11 = 1;
    R12 = 1; T12 = 1; % Trọng số cho u2, v2 trong hàm mục tiêu của 1
    R14 = 1; T14 = 1; % Trọng số cho u4, v4 trong hàm mục tiêu của 1
    
    R22 = 1; T22 = 1; % Của node 2
    R44 = 1; T44 = 1; % Của node 4
    
    % Tốc độ học (Learning rates) và tham số mạng NNs
    a1 = 0.005; a1_a = 0.007; a1_d = 0.005;
    S1 = 10; F1 = 10; S_bar1 = 10; F_bar1 = 10;

    % Hàm tính ma trận đạo hàm 3x2
    dphi_1 = [2*delta1(1), 0; 
              delta1(2), delta1(1); 
              0, 2*delta1(2)];
          
    dphi_2 = [2*delta2(1), 0; 
              delta2(2), delta2(1); 
              0, 2*delta2(2)];
          
    dphi_4 = [2*delta4(1), 0; 
              delta4(2), delta4(1); 
              0, 2*delta4(2)];

    %% 3. TÍNH TÍN HIỆU ĐẦU RA ACTOR & DISTURBANCE (Eq 55, 56)
    % Tính tín hiệu u1, v1 dự kiến dựa trên trọng số hiện tại
    u1_hat = -(d1 + g1) * (1/R11) * B1' * dphi_1' * W1_a;
    d1_hat = (1/gamma^2) * (d1 + g1) * (1/T11) * D1' * dphi_1' * W1_d;

    %% 4. TÍNH TOÁN CÁC BIẾN TRUNG GIAN
    % D_bar và E_bar (3x3)
    D_bar1 = dphi_1 * B1 * (1/R11) * B1' * dphi_1';
    E_bar1 = dphi_1 * D1 * (1/T11) * D1' * dphi_1';
    
    % Tính sigma_{i+N} (Lưu ý: dùng u_hat, v_hat theo đúng lý thuyết)
    sigma_1_N = dphi_1 * (A * delta1 + (d1 + g1)*B1*u1_hat - (B2*u2_hat + B4*u4_hat) ...
                          + (d1 + g1)*D1*d1_hat - (D2*d2_hat + D4*d4_hat));
                      
    m_s1 = (sigma_1_N' * sigma_1_N) + 1;
    sigma_bar_1_N = sigma_1_N / m_s1; % Vector 3x1

    %% 5. TÍNH TỔNG TỪ CÁC HÀNG XÓM (Node 2 và Node 4)
    % -- Của Node 2 --
    term_B2 = dphi_2 * B2 * (1/R22) * R12 * (1/R22) * B2' * dphi_2';
    term_D2 = dphi_2 * D2 * (1/T22) * T12 * (1/T22) * D2' * dphi_2';
    
    sum57_a_2 = (d2 + g2)^2 * W2_a' * term_B2 * W2_a;
    sum57_d_2 = (d2 + g2)^2 * W2_d' * term_D2 * W2_d;
    sum58_a_2 = (d2 + g2)^2 * term_B2 * W2_a .* (sigma_bar_1_N' * W2_c / m_s1);
    sum59_d_2 = (d2 + g2)^2 * term_D2 * W2_d .* (sigma_bar_1_N' * W2_c / m_s1);
    
    % -- Của Node 4 --
    term_B4 = dphi_4 * B4 * (1/R44) * R14 * (1/R44) * B4' * dphi_4';
    term_D4 = dphi_4 * D4 * (1/T44) * T14 * (1/T44) * D4' * dphi_4';
    
    sum57_a_4 = (d4 + g4)^2 * W4_a' * term_B4 * W4_a;
    sum57_d_4 = (d4 + g4)^2 * W4_d' * term_D4 * W4_d;
    sum58_a_4 = (d4 + g4)^2 * term_B4 * W4_a .* (sigma_bar_1_N' * W4_c / m_s1);
    sum59_d_4 = (d4 + g4)^2 * term_D4 * W4_d .* (sigma_bar_1_N' * W4_c / m_s1);
    
    % Gộp tổng
    sum57_actor = sum57_a_2 + sum57_a_4; % Vô hướng
    sum57_dist  = sum57_d_2 + sum57_d_4; % Vô hướng
    sum58_actor = sum58_a_2 + sum58_a_4; % Vector 3x1
    sum59_dist  = sum59_d_2 + sum59_d_4; % Vector 3x1

    %% 6. LUẬT CẬP NHẬT TRỌNG SỐ (Equations 57, 58, 59)
    % 6.1 Critic
    term1_57 = sigma_1_N' * W1_c + 0.5 * delta1' * Q11 * delta1;
    term2_57 = 0.5 * (d1 + g1)^2 * W1_a' * D_bar1 * W1_a;
    term3_57 = - (1 / (2 * gamma^2)) * (d1 + g1)^2 * W1_d' * E_bar1 * W1_d;
    term_sum_57 = 0.5 * sum57_actor - (1 / (2 * gamma^2)) * sum57_dist;
    
    gain_57 = a1 * (sigma_1_N / (m_s1^2)); % Vector 3x1
    dW1_c = - gain_57 * (term1_57 + term2_57 + term3_57 + term_sum_57);
    
    % 6.2 Actor
    % term1_58 = S1 * W1_a - F1 * W1_c;
    term1_58 = S1 * W1_a - F1 * ( W1_c) ;  % scalar
    
    term2_58 = (d1 + g1)^2 * D_bar1 * W1_a .* (sigma_bar_1_N' * W1_c / m_s1);
    dW1_a = - a1_a * (term1_58 - term2_58 - sum58_actor);
    
    % 6.3 Disturbance
    % term1_59 = S_bar1 * W1_d - F_bar1 * W1_c;
    term1_59 = S_bar1 * W1_d - F_bar1 * sigma_bar_1_N * (sigma_bar_1_N' * W1_c);

    term2_59 = (1 / gamma^2) * (d1 + g1)^2 * E_bar1 * W1_d .* (sigma_bar_1_N' * W1_c / m_s1);
    term_sum_59 = (1 / gamma^2) * sum59_dist;
    dW1_d = - a1_d * (term1_59 + term2_59 + term_sum_59);

end

== matlab function Simulink_BTL_Model_2018b/Follower 3/MATLAB Function ==
  data: W3_c input; W3_a input; W3_d input; W2_c input; W2_a input; W2_d input; u3_hat output; W4_c input; W4_a input; W4_d input; u2_hat input; u4_hat input; d2_hat input; d4_hat input; delta3 input; delta2 input; delta4 input; d3_hat output; dW3_c output; dW3_a output; dW3_d output
function [u3_hat, d3_hat, dW3_c, dW3_a, dW3_d] = Follower3_Controller(W3_c, W3_a, W3_d, W2_c, W2_a, W2_d, W4_c, W4_a, W4_d, u2_hat, u4_hat, d2_hat, d4_hat, delta3, delta2, delta4)
    % CÁC BIẾN ĐẦU VÀO TỪ SIMULINK:
    % W3_*, W2_*, W4_*: Trọng số của 3 mạng NNs của bản thân và hàng xóm (3x1)
    % u2_hat, u4_hat, d2_hat, d4_hat: Tín hiệu điều khiển/nhiễu của hàng xóm (1x1)
    % delta3, delta2, delta4: Sai số bám sát của bản thân và hàng xóm (2x1)
    u3_hat = zeros(1,1);
    d3_hat = zeros(1,1);
    dW3_c = zeros(3,1);
    dW3_a = zeros(3,1);
    dW3_d = zeros(3,1);
    %% 1. KHỞI TẠO THÔNG SỐ HỆ THỐNG VÀ ĐỒ THỊ
    % Đồ thị: N3 = {2, 4}
    d3 = 2; g3 = 0; % Node 3 KHÔNG nối với Leader
    d2 = 2; g2 = 1; % Node 2 CÓ nối với Leader
    d4 = 2; g4 = 0; % Node 4 KHÔNG nối với Leader
    
    gamma = 1; % Hệ số L2-gain
    
    % Ma trận động học
    A  = [0 0.1; -0.1 0]; 
    B2 = [2; -3]; D2 = [2; -2];
    B3 = [1; -2]; D3 = [2; -2];
    B4 = [1; -3]; D4 = [2; -3];
    
    % Ma trận trọng số chi phí (Q, R, T)
    Q33 = eye(2);
    R33 = 1; T33 = 1;
    R32 = 1; T32 = 1; % Trọng số cho u2, d2 trong hàm mục tiêu của 3
    R34 = 1; T34 = 1; % Trọng số cho u4, d4 trong hàm mục tiêu của 3
    
    R22 = 1; T22 = 1; % Của node 2
    R44 = 1; T44 = 1; % Của node 4
    
    % Tốc độ học và tham số mạng NNs
    a3 = 0.005; a3_a = 0.007; a3_d = 0.005;
    S3 = 10; F3 = 10; S_bar3 = 10; F_bar3 = 10;

    %% 2. TÍNH MA TRẬN ĐẠO HÀM (JACOBIAN) 3x2
    dphi_3 = [2*delta3(1), 0; 
              delta3(2), delta3(1); 
              0, 2*delta3(2)];
          
    dphi_2 = [2*delta2(1), 0; 
              delta2(2), delta2(1); 
              0, 2*delta2(2)];
          
    dphi_4 = [2*delta4(1), 0; 
              delta4(2), delta4(1); 
              0, 2*delta4(2)];

    %% 3. TÍNH TÍN HIỆU ĐẦU RA ACTOR & DISTURBANCE 
    u3_hat = -(d3 + g3) * (1/R33) * B3' * dphi_3' * W3_a;
    d3_hat = (1/gamma^2) * (d3 + g3) * (1/T33) * D3' * dphi_3' * W3_d;

    %% 4. TÍNH TOÁN CÁC BIẾN TRUNG GIAN (3x3)
    D_bar3 = dphi_3 * B3 * (1/R33) * B3' * dphi_3';
    E_bar3 = dphi_3 * D3 * (1/T33) * D3' * dphi_3';
    
    % Tính sigma_{i+N} 
    sigma_3_N = dphi_3 * (A * delta3 + (d3 + g3)*B3*u3_hat - (B2*u2_hat + B4*u4_hat) ...
                          + (d3 + g3)*D3*d3_hat - (D2*d2_hat + D4*d4_hat));
                      
    m_s3 = (sigma_3_N' * sigma_3_N) + 1;
    sigma_bar_3_N = sigma_3_N / m_s3; % Vector 3x1

    %% 5. TÍNH TỔNG TỪ CÁC HÀNG XÓM (Node 2 và Node 4)
    % -- Của Node 2 --
    term_B2 = dphi_2 * B2 * (1/R22) * R32 * (1/R22) * B2' * dphi_2';
    term_D2 = dphi_2 * D2 * (1/T22) * T32 * (1/T22) * D2' * dphi_2';
    
    sum57_a_2 = (d2 + g2)^2 * W2_a' * term_B2 * W2_a;
    sum57_d_2 = (d2 + g2)^2 * W2_d' * term_D2 * W2_d;
    sum58_a_2 = (d2 + g2)^2 * term_B2 * W2_a .* (sigma_bar_3_N' * W2_c / m_s3);
    sum59_d_2 = (d2 + g2)^2 * term_D2 * W2_d .* (sigma_bar_3_N' * W2_c / m_s3);
    
    % -- Của Node 4 --
    term_B4 = dphi_4 * B4 * (1/R44) * R34 * (1/R44) * B4' * dphi_4';
    term_D4 = dphi_4 * D4 * (1/T44) * T34 * (1/T44) * D4' * dphi_4';
    
    sum57_a_4 = (d4 + g4)^2 * W4_a' * term_B4 * W4_a;
    sum57_d_4 = (d4 + g4)^2 * W4_d' * term_D4 * W4_d;
    sum58_a_4 = (d4 + g4)^2 * term_B4 * W4_a .* (sigma_bar_3_N' * W4_c / m_s3);
    sum59_d_4 = (d4 + g4)^2 * term_D4 * W4_d .* (sigma_bar_3_N' * W4_c / m_s3);
    
    % Gộp tổng
    sum57_actor = sum57_a_2 + sum57_a_4; 
    sum57_dist  = sum57_d_2 + sum57_d_4; 
    sum58_actor = sum58_a_2 + sum58_a_4; 
    sum59_dist  = sum59_d_2 + sum59_d_4; 

    %% 6. LUẬT CẬP NHẬT TRỌNG SỐ
    % 6.1 Critic
    term1_57 = sigma_3_N' * W3_c + 0.5 * delta3' * Q33 * delta3;
    term2_57 = 0.5 * (d3 + g3)^2 * W3_a' * D_bar3 * W3_a;
    term3_57 = - (1 / (2 * gamma^2)) * (d3 + g3)^2 * W3_d' * E_bar3 * W3_d;
    term_sum_57 = 0.5 * sum57_actor - (1 / (2 * gamma^2)) * sum57_dist;
    
    gain_57 = a3 * (sigma_3_N / (m_s3^2)); 
    dW3_c = - gain_57 * (term1_57 + term2_57 + term3_57 + term_sum_57);
    
    % 6.2 Actor
    % term1_58 = S3 * W3_a - F3 * W3_c;
    term1_58 = S3 * W3_a - F3 * ( W3_c) ;  % scalar
    term2_58 = (d3 + g3)^2 * D_bar3 * W3_a .* (sigma_bar_3_N' * W3_c / m_s3);
    dW3_a = - a3_a * (term1_58 - term2_58 - sum58_actor);
    
    % 6.3 Disturbance
    % term1_59 = S_bar3 * W3_d - F_bar3 * W3_c;
    term1_59 = S_bar3 * W3_d - F_bar3 * sigma_bar_3_N * (sigma_bar_3_N' * W3_c);

    term2_59 = (1 / gamma^2) * (d3 + g3)^2 * E_bar3 * W3_d .* (sigma_bar_3_N' * W3_c / m_s3);
    term_sum_59 = (1 / gamma^2) * sum59_dist;
    dW3_d = - a3_d * (term1_59 + term2_59 + term_sum_59);
end

== matlab function Simulink_BTL_Model_2018b/Follower 4/MATLAB Function ==
  data: W4_c input; W4_a input; W4_d input; W1_c input; W1_a input; W1_d input; W3_c input; W3_a input; W3_d input; u4_hat output; u1_hat input; u3_hat input; d1_hat input; d3_hat input; delta4 input; delta1 input; delta3 input; d4_hat output; dW4_c output; dW4_a output; dW4_d output
function [u4_hat, d4_hat, dW4_c, dW4_a, dW4_d] = Follower4_Controller(W4_c, W4_a, W4_d, W1_c, W1_a, W1_d, W3_c, W3_a, W3_d, u1_hat, u3_hat, d1_hat, d3_hat, delta4, delta1, delta3)
    % CÁC BIẾN ĐẦU VÀO TỪ SIMULINK:
    % W4_*, W1_*, W3_*: Trọng số của 3 mạng NNs của bản thân và hàng xóm (3x1)
    % u1_hat, u3_hat, d1_hat, d3_hat: Tín hiệu điều khiển/nhiễu của hàng xóm (1x1)
    % delta4, delta1, delta3: Sai số bám sát của bản thân và hàng xóm (2x1)
    u4_hat = zeros(1,1);
    d4_hat = zeros(1,1);
    dW4_c = zeros(3,1);
    dW4_a = zeros(3,1);
    dW4_d = zeros(3,1);
    %% 1. KHỞI TẠO THÔNG SỐ HỆ THỐNG VÀ ĐỒ THỊ
    % Đồ thị: N4 = {1, 3}
    d4 = 2; g4 = 0; % Node 4 KHÔNG nối với Leader
    d1 = 2; g1 = 1; % Node 1 CÓ nối với Leader
    d3 = 2; g3 = 0; % Node 3 KHÔNG nối với Leader
    
    gamma = 1; % Hệ số L2-gain
    
    % Ma trận động học
    A  = [0 0.1; -0.1 0]; 
    B1 = [2; -1]; D1 = [2; -1];
    B3 = [1; -2]; D3 = [2; -2];
    B4 = [1; -3]; D4 = [2; -3];
    
    % Ma trận trọng số chi phí (Q, R, T)
    Q44 = eye(2);
    R44 = 1; T44 = 1;
    R41 = 1; T41 = 1; % Trọng số cho u1, d1 trong hàm mục tiêu của 4
    R43 = 1; T43 = 1; % Trọng số cho u3, d3 trong hàm mục tiêu của 4
    
    R11 = 1; T11 = 1; % Của node 1
    R33 = 1; T33 = 1; % Của node 3
    
    % Tốc độ học và tham số mạng NNs
    a4 = 0.005; a4_a = 0.007; a4_d = 0.005;
    S4 = 10; F4 =10; S_bar4 = 10; F_bar4 = 10;

    %% 2. TÍNH MA TRẬN ĐẠO HÀM (JACOBIAN) 3x2
    dphi_4 = [2*delta4(1), 0; 
              delta4(2), delta4(1); 
              0, 2*delta4(2)];
          
    dphi_1 = [2*delta1(1), 0; 
              delta1(2), delta1(1); 
              0, 2*delta1(2)];
          
    dphi_3 = [2*delta3(1), 0; 
              delta3(2), delta3(1); 
              0, 2*delta3(2)];

    %% 3. TÍNH TÍN HIỆU ĐẦU RA ACTOR & DISTURBANCE 
    u4_hat = -(d4 + g4) * (1/R44) * B4' * dphi_4' * W4_a;
    d4_hat = (1/gamma^2) * (d4 + g4) * (1/T44) * D4' * dphi_4' * W4_d;

    %% 4. TÍNH TOÁN CÁC BIẾN TRUNG GIAN (3x3)
    D_bar4 = dphi_4 * B4 * (1/R44) * B4' * dphi_4';
    E_bar4 = dphi_4 * D4 * (1/T44) * D4' * dphi_4';
    
    % Tính sigma_{i+N} 
    sigma_4_N = dphi_4 * (A * delta4 + (d4 + g4)*B4*u4_hat - (B1*u1_hat + B3*u3_hat) ...
                          + (d4 + g4)*D4*d4_hat - (D1*d1_hat + D3*d3_hat));
                      
    m_s4 = (sigma_4_N' * sigma_4_N) + 1;
    sigma_bar_4_N = sigma_4_N / m_s4; % Vector 3x1

    %% 5. TÍNH TỔNG TỪ CÁC HÀNG XÓM (Node 1 và Node 3)
    % -- Của Node 1 --
    term_B1 = dphi_1 * B1 * (1/R11) * R41 * (1/R11) * B1' * dphi_1';
    term_D1 = dphi_1 * D1 * (1/T11) * T41 * (1/T11) * D1' * dphi_1';
    
    sum57_a_1 = (d1 + g1)^2 * W1_a' * term_B1 * W1_a;
    sum57_d_1 = (d1 + g1)^2 * W1_d' * term_D1 * W1_d;
    sum58_a_1 = (d1 + g1)^2 * term_B1 * W1_a .* (sigma_bar_4_N' * W1_c / m_s4);
    sum59_d_1 = (d1 + g1)^2 * term_D1 * W1_d .* (sigma_bar_4_N' * W1_c / m_s4);
    
    % -- Của Node 3 --
    term_B3 = dphi_3 * B3 * (1/R33) * R43 * (1/R33) * B3' * dphi_3';
    term_D3 = dphi_3 * D3 * (1/T33) * T43 * (1/T33) * D3' * dphi_3';
    
    sum57_a_3 = (d3 + g3)^2 * W3_a' * term_B3 * W3_a;
    sum57_d_3 = (d3 + g3)^2 * W3_d' * term_D3 * W3_d;
    sum58_a_3 = (d3 + g3)^2 * term_B3 * W3_a .* (sigma_bar_4_N' * W3_c / m_s4);
    sum59_d_3 = (d3 + g3)^2 * term_D3 * W3_d .* (sigma_bar_4_N' * W3_c / m_s4);
    
    % Gộp tổng
    sum57_actor = sum57_a_1 + sum57_a_3; 
    sum57_dist  = sum57_d_1 + sum57_d_3; 
    sum58_actor = sum58_a_1 + sum58_a_3; 
    sum59_dist  = sum59_d_1 + sum59_d_3; 

    %% 6. LUẬT CẬP NHẬT TRỌNG SỐ
    % 6.1 Critic
    term1_57 = sigma_4_N' * W4_c + 0.5 * delta4' * Q44 * delta4;
    term2_57 = 0.5 * (d4 + g4)^2 * W4_a' * D_bar4 * W4_a;
    term3_57 = - (1 / (2 * gamma^2)) * (d4 + g4)^2 * W4_d' * E_bar4 * W4_d;
    term_sum_57 = 0.5 * sum57_actor - (1 / (2 * gamma^2)) * sum57_dist;
    
    gain_57 = a4 * (sigma_4_N / (m_s4^2)); 
    dW4_c = - gain_57 * (term1_57 + term2_57 + term3_57 + term_sum_57);
    
    % 6.2 Actor
    % term1_58 = S4 * W4_a - F4 * W4_c;
    term1_58 = S4 * W4_a - F4 * ( W4_c) ;  % scalar

    term2_58 = (d4 + g4)^2 * D_bar4 * W4_a .* (sigma_bar_4_N' * W4_c / m_s4);
    dW4_a = - a4_a * (term1_58 - term2_58 - sum58_actor);
    
    % 6.3 Disturbance
    % term1_59 = S_bar4 * W4_d - F_bar4 * W4_c;
    term1_59 = S_bar4 * W4_d - F_bar4 * sigma_bar_4_N * (sigma_bar_4_N' * W4_c);

    term2_59 = (1 / gamma^2) * (d4 + g4)^2 * E_bar4 * W4_d .* (sigma_bar_4_N' * W4_c / m_s4);
    term_sum_59 = (1 / gamma^2) * sum59_dist;
    dW4_d = - a4_d * (term1_59 + term2_59 + term_sum_59);
end
